simulink model "train_dynamics"  (R2025a)
settings: Solver=FixedStepAuto  StartTime=0.0  StopTime=10.0  FixedStep=0.05  RelTol=1e-3
values from neighbouring files (symbols this model uses):
  brake_force = 90000.0    [train_dynamics.sldd]
  gearRatio = 16.0    [train_dynamics.sldd]
  massPerCar = 27272.727272727272    [train_dynamics.sldd]
  massPerTug = 27272.727272727272    [train_dynamics.sldd]
  maxTorque = 260.0    [train_dynamics.sldd]
  nCars = 0.0    [train_dynamics.sldd]
  nMotorsPerTug = 1.0    [train_dynamics.sldd]
  nTugVolts = 1.0    [train_dynamics.sldd]
  pInit = 0.0    [train_dynamics.sldd]
  vInit = 0.0    [train_dynamics.sldd]
undefined symbols (not defined in the file or in its folder): DiscIntNeverNeededParam
libraries: simulink_extras x1
settings Model: DataDictionary=train_dynamics.sldd  Creator=samki  LastModifiedBy=adam
settings OptimizationCC: DefaultParameterBehavior=Inlined  UseDivisionForNetSlopeComputation=on  GainParamInheritBuiltInType=on  UseFloatMulNetSlope=on  InlineInvariantSignals=on  EnhancedBackFolding=on  PassReuseOutputArgsAs=Individual arguments  ZeroExternalMemoryAtStartup=off  ZeroInternalMemoryAtStartup=off  EfficientFloat2IntCast=on  OptimizeBlockOrder=speed  DifferentSizesBufferReuse=on  OptimizationCustomize=off  EfficientTunableParamExpr=on
settings DebuggingCC: SignalInfNanChecking=warning  IntegerOverflowMsg=error  ParameterTunabilityLossMsg=error  AssertControl=DisableAll  SFUndirectedBroadcastEventsDiag=error
settings HardwareCC: ProdLongLongMode=on
settings SFSimCC: CompileTimeRecursionLimit=0.0  EnableRuntimeRecursion=off  MATLABDynamicMemAlloc=off
settings RTWCC: SystemTargetFile=ert.tlc  PackageGeneratedCodeAndArtifacts=on  TemplateMakefile=ert_default_tmf  Toolchain=GNU gcc/g++ | gmake (64-bit Linux)  GPUComputeCapability=3.5  Description=Embedded Coder
settings CodeAppCC: ForceParamTrailComments=on  IgnoreCustomStorageClasses=off  OperatorAnnotations=on  SimulinkDataObjDesc=on  SFDataObjDesc=on  InsertBlockDesc=on
settings ERTTargetCC: ExtModeTransport=0.0  ExtModeStaticAlloc=off  ExtModeMexFile=ext_comm  ExtModeIntrfLevel=Level1  ERTCustomFileTemplate=example_file_process.tlc  TargetLangStandard=C99 (ISO)  GenerateSampleERTMain=on

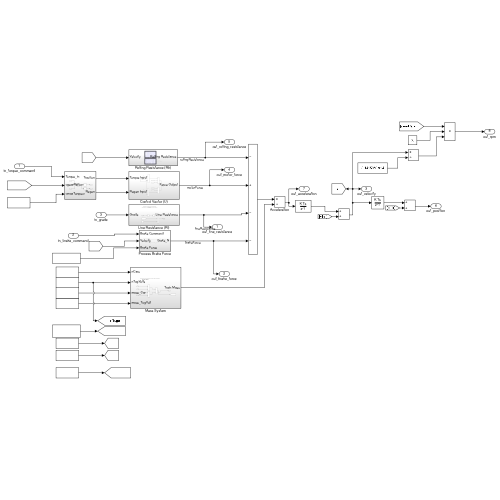
[thumbnail: Simulink's stored preview of the top-level diagram]
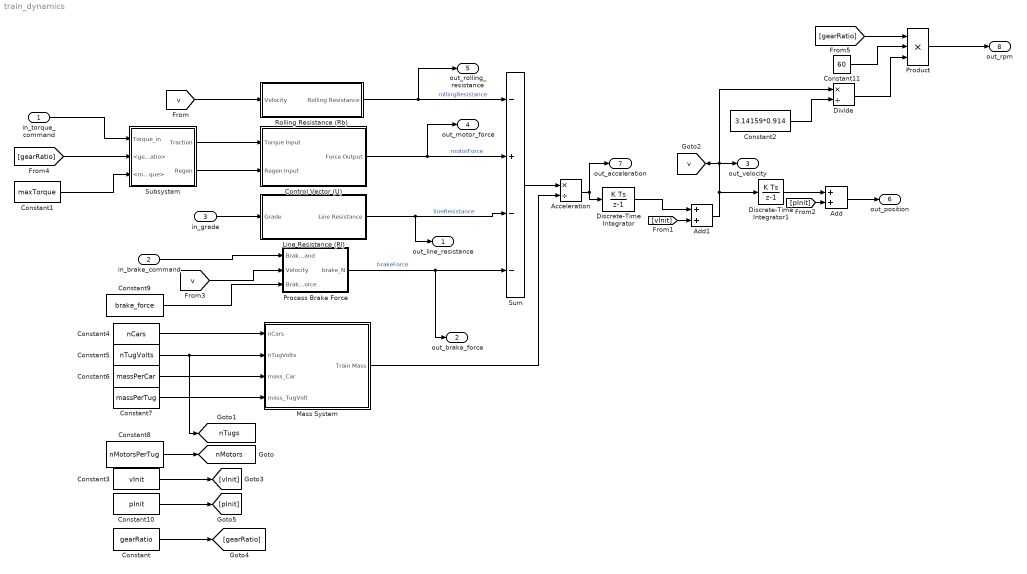
== system train_dynamics ==
  in_torque_command : Inport
  in_brake_command : Inport  Port=2
  in_grade : Inport  Port=3
  Acceleration : Product  Inputs=*/
  Add : Sum
  Add1 : Sum
  Constant : Constant  Value=gearRatio
  Constant1 : Constant  Value=maxTorque
  Constant10 : Constant  Value=pInit
  Constant11 : Constant  Value=60
  Constant2 : Constant  Value=3.14159*0.914
  Constant3 : Constant  Value=vInit
  Constant4 : Constant  Value=nCars
  Constant5 : Constant  Value=nTugVolts
  Constant6 : Constant  Value=massPerCar
  Constant7 : Constant  Value=massPerTug
  Constant8 : Constant  Value=nMotorsPerTug
  Constant9 : Constant  Value=brake_force
  Control Vector (U) : Subsystem
  Discrete-Time Integrator : DiscreteIntegrator  SampleTime=-1  LowerSaturationLimit=0  ICPrevOutput=DiscIntNeverNeededParam  ICPrevScaledInput=DiscIntNeverNeededParam
  Discrete-Time Integrator1 : DiscreteIntegrator  SampleTime=-1  ICPrevOutput=DiscIntNeverNeededParam  ICPrevScaledInput=DiscIntNeverNeededParam
  Divide : Product  Inputs=*/
  Line Resistance (Rl) : Subsystem
  Mass System : Subsystem
  Process Brake Force : Subsystem
  Product : Product  Inputs=3
  Rolling Resistance (Rb) : Subsystem
  Subsystem : Subsystem
  Sum : Sum  Inputs=-+--
  out_line_resistance : Outport
  out_brake_force : Outport  Port=2
  out_velocity : Outport  Port=3
  out_motor_force : Outport  Port=4
  out_rolling_resistance : Outport  Port=5
  out_position : Outport  Port=6
  out_acceleration : Outport  Port=7
  out_rpm : Outport  Port=8
  tag scope: nMotors=global, nTugs=global, v=global
  wires:
  Control Vector (U)/1(Force Output) -> Sum/2, out_motor_force/1  "motorForce"
  Rolling Resistance (Rb)/1(Rolling Resistance) -> Sum/1, out_rolling_resistance/1  "rollingResistance"
  Acceleration/1 -> Discrete-Time Integrator/1, out_acceleration/1
  Line Resistance (Rl)/1(Line Resistance) -> Sum/3, out_line_resistance/1  "lineResistance"
  Mass System/1(Train Mass) -> Acceleration/2
  Sum/1 -> Acceleration/1
  Add1/1 -> Divide/1, out_velocity/1, [v], Discrete-Time Integrator1/1
  Process Brake Force/1(brake_N) -> Sum/4, out_brake_force/1  "brakeForce"
  in_brake_command/1 -> Process Brake Force/1(Brake Command)
  in_torque_command/1 -> Subsystem/1(Torque_in)
  Subsystem/1(Traction) -> Control Vector (U)/1(Torque Input)
  Subsystem/2(Regen) -> Control Vector (U)/2(Regen Input)
  Constant1/1 -> Subsystem/3(<maxTorque>)
  in_grade/1 -> Line Resistance (Rl)/1(Grade)
  Constant3/1 -> [vInit]
  Constant4/1 -> Mass System/1(nCars)
  Constant5/1 -> [nTugs], Mass System/2(nTugVolts)
  Constant6/1 -> Mass System/3(mass_Car)
  Constant7/1 -> Mass System/4(mass_TugVolt)
  Constant8/1 -> [nMotors]
  Constant9/1 -> Process Brake Force/3(Brake Force)
  Constant10/1 -> [pInit]
  [v] -> Process Brake Force/2(Velocity)
  [v] -> Rolling Resistance (Rb)/1(Velocity)
  Constant/1 -> [gearRatio]
  [gearRatio] -> Subsystem/2(<gearRatio>)
  [gearRatio] -> Product/1
  Constant2/1 -> Divide/2
  Divide/1 -> Product/3
  Product/1 -> out_rpm/1
  Constant11/1 -> Product/2
  Discrete-Time Integrator1/1 -> Add/1
  [pInit] -> Add/2
  Add/1 -> out_position/1
  [vInit] -> Add1/2
  Discrete-Time Integrator/1 -> Add1/1

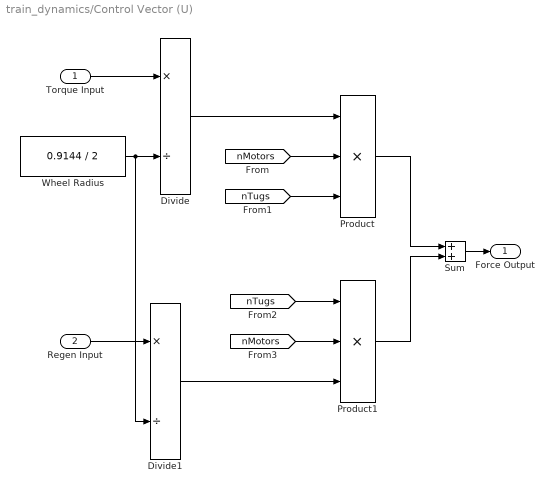
== system train_dynamics/Control Vector (U) ==
  Torque Input : Inport
  Regen Input : Inport  Port=2
  Divide : Product  Inputs=*/
  Divide1 : Product  Inputs=*/
  Product : Product  Inputs=3
  Product1 : Product  Inputs=3
  Sum : Sum
  Wheel Radius : Constant  Value=0.9144 / 2
  Force Output : Outport
  wires:
  Sum/1 -> Force Output/1
  Product/1 -> Sum/1
  Product1/1 -> Sum/2
  Regen Input/1 -> Divide1/1
  Divide1/1 -> Product1/3
  [nMotors] -> Product1/2
  [nTugs] -> Product1/1
  Divide/1 -> Product/1
  Torque Input/1 -> Divide/1
  Wheel Radius/1 -> Divide/2, Divide1/2
  [nTugs] -> Product/3
  [nMotors] -> Product/2

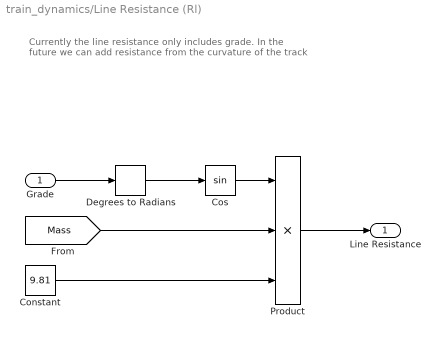
== system train_dynamics/Line Resistance (Rl) ==
  note: Currently the line resistance only includes grade.
      | In the future we can add resistance from the curvature of
      | the track
  Grade : Inport
  Constant : Constant  Value=9.81
  Cos : Trigonometry
  Degrees to Radians : simulink_extras/Transformations/Degrees to Radians
  Product : Product  Inputs=3
  Line Resistance : Outport
  wires:
  Degrees to Radians/1 -> Cos/1
  [Mass] -> Product/2
  Cos/1 -> Product/1
  Constant/1 -> Product/3
  Product/1 -> Line Resistance/1
  Grade/1 -> Degrees to Radians/1

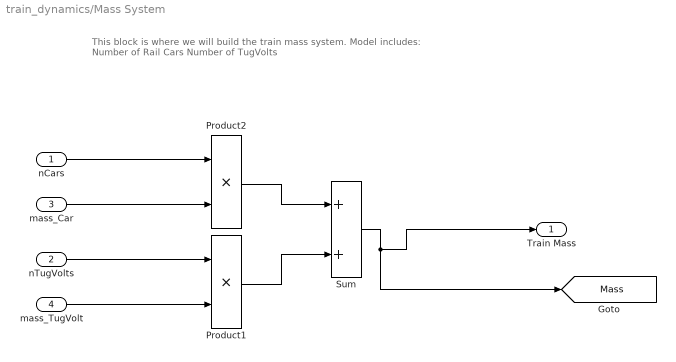
== system train_dynamics/Mass System ==
  note: This block is where we will build the train mass system. Model includes:
      | Number of Rail Cars
      | Number of TugVolts
  nCars : Inport
  nTugVolts : Inport  Port=2
  mass_Car : Inport  Port=3
  mass_TugVolt : Inport  Port=4
  Product1 : Product
  Product2 : Product
  Sum : Sum
  Train Mass : Outport
  tag scope: Mass=global
  wires:
  Product1/1 -> Sum/2
  nTugVolts/1 -> Product1/1
  mass_TugVolt/1 -> Product1/2
  Product2/1 -> Sum/1
  nCars/1 -> Product2/1
  mass_Car/1 -> Product2/2
  Sum/1 -> Train Mass/1, [Mass]

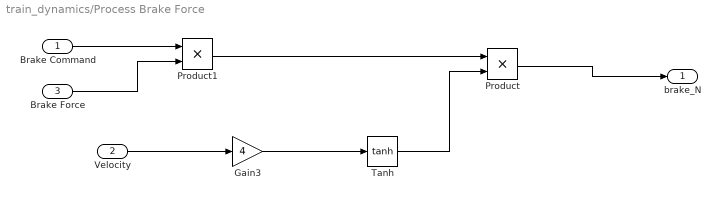
== system train_dynamics/Process Brake Force ==
  Brake Command : Inport
  Velocity : Inport  Port=2
  Brake Force : Inport  Port=3
  Gain3 : Gain  Gain=4
  Product : Product
  Product1 : Product
  Tanh : Trigonometry  Operator=tanh
  brake_N : Outport
  wires:
  Velocity/1 -> Gain3/1
  Gain3/1 -> Tanh/1
  Tanh/1 -> Product/2
  Brake Command/1 -> Product1/1
  Brake Force/1 -> Product1/2
  Product/1 -> brake_N/1
  Product1/1 -> Product/1

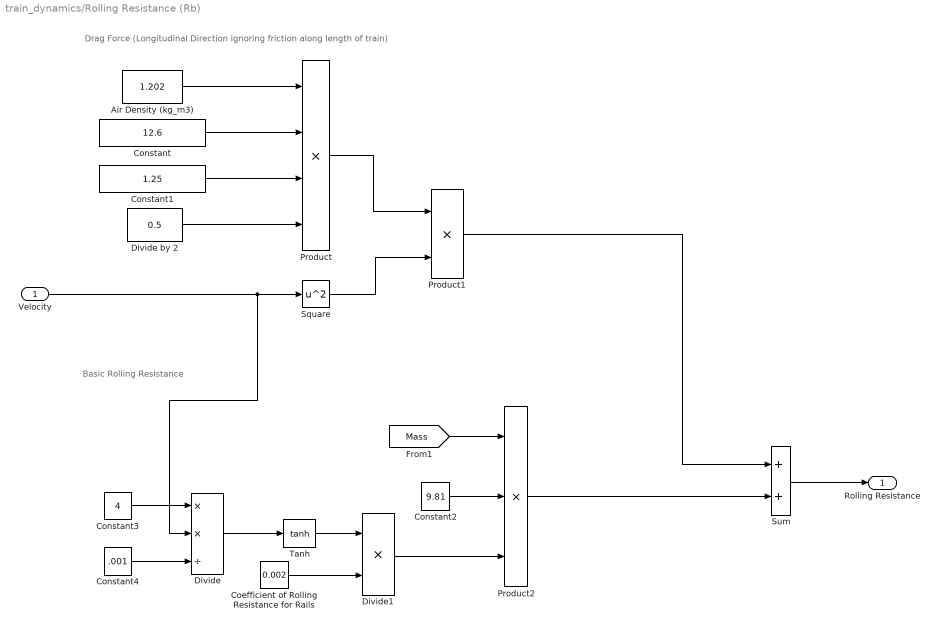
== system train_dynamics/Rolling Resistance (Rb) ==
  note: Basic Rolling Resistance
  note: Drag Force (Longitudinal Direction ignoring friction along length of train)
  Velocity : Inport
  Air Density (kg_m3) : Constant  Value=1.202
  Coefficient of Rolling Resistance for Rails : Constant  Value=0.002
  Constant : Constant  Value=12.6
  Constant1 : Constant  Value=1.25
  Constant2 : Constant  Value=9.81
  Constant3 : Constant  Value=4
  Constant4 : Constant  Value=.001
  Divide : Product  Inputs=**/
  Divide by 2 : Constant  Value=0.5
  Divide1 : Product  Inputs=**
  Product : Product  Inputs=4
  Product1 : Product
  Product2 : Product  Inputs=3
  Square : Math  Operator=square
  Sum : Sum
  Tanh : Trigonometry  Operator=tanh
  Rolling Resistance : Outport
  wires:
  Product2/1 -> Sum/2
  Sum/1 -> Rolling Resistance/1
  Product1/1 -> Sum/1
  Constant1/1 -> Product/3
  Velocity/1 -> Divide/2, Square/1
  Constant/1 -> Product/2
  Square/1 -> Product1/2
  Air Density (kg_m3)/1 -> Product/1
  Product/1 -> Product1/1
  Divide by 2/1 -> Product/4
  [Mass] -> Product2/1
  Constant2/1 -> Product2/2
  Constant4/1 -> Divide/3
  Constant3/1 -> Divide/1
  Divide/1 -> Tanh/1
  Tanh/1 -> Divide1/1
  Coefficient of Rolling Resistance for Rails/1 -> Divide1/2
  Divide1/1 -> Product2/3

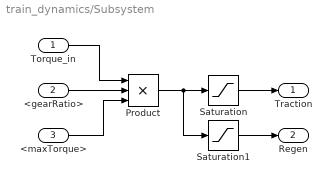
== system train_dynamics/Subsystem ==
  Torque_in : Inport
  <gearRatio> : Inport  Port=2
  <maxTorque> : Inport  Port=3
  Product : Product  Inputs=3
  Saturation : Saturate  UpperLimit=10000  LowerLimit=0
  Saturation1 : Saturate  UpperLimit=0  LowerLimit=-10000
  Traction : Outport
  Regen : Outport  Port=2
  wires:
  Product/1 -> Saturation1/1, Saturation/1
  Torque_in/1 -> Product/1
  <gearRatio>/1 -> Product/2
  Saturation1/1 -> Regen/1
  <maxTorque>/1 -> Product/3
  Saturation/1 -> Traction/1
